simulink model "QuadPIDv2"  (R2024b)
settings: Solver=VariableStepAuto  StartTime=0.0  StopTime=50  RelTol=1e-3
libraries: aerolibutil x9, matrix_library x2, sharedutil x2, sharedtransform x1, simulink_extras x1
settings Model: Creator=Jorge  LastModifiedBy=Jorge

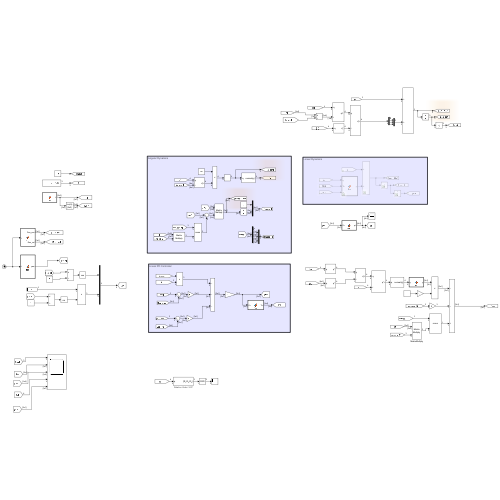
[thumbnail: Simulink's stored preview of the top-level diagram]
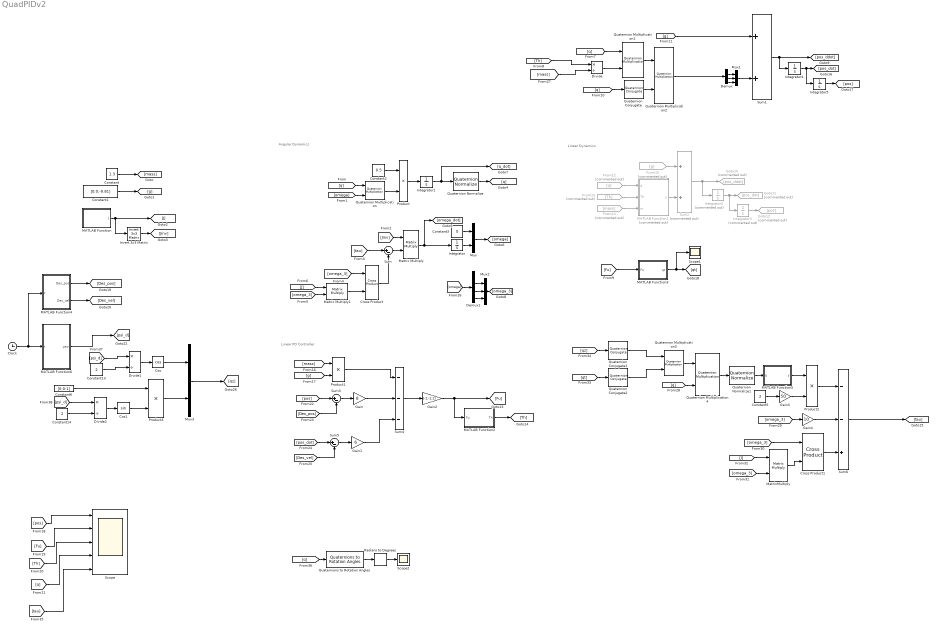
== system QuadPIDv2 ==
  note: Linear PD Controller
  note: Linear Dynamics
  note: Angular Dynamics
  Clock : Clock
  Constant : Constant  Value=1.3
  Constant1 : Constant  Value=[0;0;-9.81]
  Constant13 : Constant  Value=2
  Constant14 : Constant  Value=2
  Constant2 : Constant  Value=0.5
  Constant3 : Constant  Value=0
  Constant5 : Constant  Value=2
  Constant6 : Constant  Value=[0;0;1]
  Cos : Trigonometry  Operator=cos
  Cos1 : Trigonometry
  Cross Product : matrix_library/Cross Product
  Cross Product1 : matrix_library/Cross Product
  Demux : Demux
  Demux1 : Demux
  Divide : Product  Inputs=*/
  Divide1 : Product  Inputs=*/
  Divide2 : Product  Inputs=*/
  From12 : From  Commented=on  GotoTag=q
  From13 : From  Commented=on  GotoTag=Th
  From14 : From  Commented=on  GotoTag=mass
  From15 : From  Commented=on  GotoTag=g
  Gain : Gain  Gain=8
  Gain1 : Gain  Gain=6
  Gain2 : Gain  Gain=[-1;-1;1]
  Gain3 : Gain  Gain=50
  Gain4 : Gain  Gain=10
  Goto10 : Goto  Commented=on  GotoTag=pos_ddot
  Goto11 : Goto  Commented=on  GotoTag=pos_dot
  Goto12 : Goto  Commented=on  GotoTag=pos
  Integrator : Integrator  InitialCondition=[0;0;0]
  Integrator1 : Integrator  InitialCondition=[1;0;0;0]
  Integrator2 : Integrator  Commented=on
  Integrator3 : Integrator  Commented=on
  Integrator4 : Integrator  InitialCondition=[0;0;0]
  Integrator5 : Integrator  InitialCondition=[0;0;0]
  Invert 3x3 Matrix : aerolibutil/Invert  3x3 Matrix
  MATLAB Function : MATLAB Function  TreatAsAtomicUnit=on
  MATLAB Function1 : MATLAB Function  Commented=on  TreatAsAtomicUnit=on
  MATLAB Function2 : MATLAB Function  TreatAsAtomicUnit=on
  MATLAB Function3 : MATLAB Function  TreatAsAtomicUnit=on
  MATLAB Function4 : MATLAB Function  TreatAsAtomicUnit=on
  MATLAB Function5 : MATLAB Function  TreatAsAtomicUnit=on
  MATLAB Function6 : MATLAB Function  TreatAsAtomicUnit=on
  Matrix Multiply : Product  Multiplication=Matrix(*)
  Matrix Multiply1 : Product  Multiplication=Matrix(*)
  MatrixMultiply : Product  Multiplication=Matrix(*)
  Mux : Mux  Inputs=2
  Mux1 : Mux  Inputs=3
  Mux2 : Mux  Inputs=3
  Mux3 : Mux  Inputs=2
  Product{,1..3} (4 alike) : Product
  Quaternion Conjugate : aerolibutil/Quaternion Conjugate
  Quaternion Conjugate1 : aerolibutil/Quaternion Conjugate
  Quaternion Conjugate2 : aerolibutil/Quaternion Conjugate
  Quaternion Multiplication{,1..4} (5 alike) : aerolibutil/Quaternion Multiplication
  Quaternion Normalize : sharedutil/Quaternion Normalize  aMode=aMode
  Quaternion Normalize1 : sharedutil/Quaternion Normalize  aMode=aMode
  Quaternions to Rotation Angles : sharedtransform/Quaternions to Rotation Angles  rotationOrder=XYZ  aMode=aMode
  Radians to Degrees : simulink_extras/Transformations/Radians to Degrees
  Scope : Scope  NumInputPorts=5
  Scope1 : Scope
  Scope2 : Scope
  Sum : Sum  Inputs=|+-
  Sum1 : Sum
  Sum2 : Sum  Commented=on
  Sum3 : Sum  Inputs=|+-
  Sum4 : Sum  Inputs=---
  Sum5 : Sum  Inputs=|+-
  Sum6 : Sum  Inputs=--+
  wires:
  Constant/1 -> [mass]
  Constant1/1 -> [g]
  MATLAB Function/1(J) -> [J], Invert 3x3 Matrix/1
  Invert 3x3 Matrix/1 -> [Jinv]
  Constant2/1 -> Product/1
  [q] -> Quaternion Multiplication/1
  [omega] -> Quaternion Multiplication/2
  Quaternion Multiplication/1 -> Product/2
  Product/1 -> Integrator1/1
  Integrator1/1 -> Quaternion Normalize/1, [q_dot]
  [Jinv] -> Matrix Multiply/1
  Matrix Multiply1/1 -> Cross Product/2
  [omega_3] -> Matrix Multiply1/2
  [J] -> Matrix Multiply1/1
  [omega_3] -> Cross Product/1
  [tau] -> Sum/1
  Cross Product/1 -> Sum/2
  Sum/1 -> Matrix Multiply/2
  Matrix Multiply/1 -> Integrator/1, [omega_dot]
  Constant3/1 -> Mux/1
  Integrator/1 -> Mux/2
  Mux/1 -> [omega]
  Quaternion Normalize/1 -> [q]
  [q] -> Quaternion Multiplication1/1
  [q] -> Quaternion Conjugate/1
  Quaternion Multiplication1/1 -> Quaternion Multiplication2/1
  Quaternion Conjugate/1 -> Quaternion Multiplication2/2
  [g] -> Sum1/1
  From12/1 -> MATLAB Function1/1(q)
  From13/1 -> MATLAB Function1/2(Th)
  From14/1 -> MATLAB Function1/3(m)
  MATLAB Function1/1(y) -> Sum2/2
  Sum2/1 -> Integrator2/1, Goto10/1
  Integrator2/1 -> Integrator3/1, Goto11/1
  Integrator3/1 -> Goto12/1
  From15/1 -> Sum2/1
  [g] -> Product1/2
  Demux/2 -> Mux1/1
  Demux/3 -> Mux1/2
  Demux/4 -> Mux1/3
  Mux1/1 -> Sum1/2
  [pos] -> Scope/1
  [Fu] -> Scope/2
  [Th] -> Scope/3
  [q] -> Scope/4
  Integrator4/1 -> [pos_dot], Integrator5/1
  Integrator5/1 -> [pos]
  Sum4/1 -> Gain2/1
  Product1/1 -> Sum4/1
  MATLAB Function2/1(Th) -> [Th]
  [mass] -> Product1/1
  [Fu] -> MATLAB Function3/1(Fu)
  MATLAB Function3/1(qt) -> Scope1/1, [qt]
  MATLAB Function4/1(Des_pos) -> [Des_pos]
  MATLAB Function4/2(Des_vel) -> [Des_vel]
  [pos] -> Sum3/1
  [Des_pos] -> Sum3/2
  Sum3/1 -> Gain/1
  Gain/1 -> Sum4/2
  Sum5/1 -> Gain1/1
  [pos_dot] -> Sum5/1
  Gain1/1 -> Sum4/3
  [Des_vel] -> Sum5/2
  Gain2/1 -> MATLAB Function2/1(Fu), [Fu]
  [qz] -> Quaternion Conjugate1/1
  [qt] -> Quaternion Conjugate2/1
  Quaternion Multiplication3/1 -> Quaternion Multiplication4/1
  [q] -> Quaternion Multiplication4/2
  Quaternion Multiplication4/1 -> Quaternion Normalize1/1
  Constant5/1 -> Gain3/1
  Gain3/1 -> Product2/2
  MATLAB Function5/1(y) -> Product2/1
  [omega_3] -> Gain4/1
  Product2/1 -> Sum6/1
  Gain4/1 -> Sum6/2
  [omega_3] -> Cross Product1/1
  [J] -> MatrixMultiply/1
  MatrixMultiply/1 -> Cross Product1/2
  [omega_3] -> MatrixMultiply/2
  Cross Product1/1 -> Sum6/3
  Quaternion Conjugate1/1 -> Quaternion Multiplication3/1
  Quaternion Conjugate2/1 -> Quaternion Multiplication3/2
  Mux2/1 -> [omega_3]
  Demux1/3 -> Mux2/2
  Demux1/2 -> Mux2/1
  Demux1/4 -> Mux2/3
  [omega] -> Demux1/1
  Quaternion Normalize1/1 -> MATLAB Function5/1(q)
  Divide/1 -> Quaternion Multiplication1/2
  [Th] -> Divide/1
  [mass] -> Divide/2
  Quaternion Multiplication2/1 -> Demux/1
  Mux3/1 -> [qz]
  Cos/1 -> Mux3/1
  Constant14/1 -> Divide2/2
  Clock/1 -> MATLAB Function4/1(t), MATLAB Function6/1(t)
  [psi_d] -> Divide1/1
  Divide1/1 -> Cos/1
  [psi_d] -> Divide2/1
  Product3/1 -> Mux3/2
  Divide2/1 -> Cos1/1
  Constant13/1 -> Divide1/2
  Cos1/1 -> Product3/2
  Constant6/1 -> Product3/1
  MATLAB Function6/1(yaw) -> [psi_d]
  [tau] -> Scope/5
  [q] -> Quaternions to Rotation Angles/1
  Quaternions to Rotation Angles/1 -> Radians to Degrees/1
  Radians to Degrees/1 -> Scope2/1
  Sum6/1 -> [tau]
  Sum1/1 -> Integrator4/1, [pos_ddot]

== matlab function QuadPIDv2/MATLAB Function ==
  data: J output
function J = fcn()

Jxx = 0.177;
Jyy = 0.177;
Jzz = 0.354; 

J = diag([Jxx,Jyy,Jzz]);

== matlab function QuadPIDv2/MATLAB Function2 ==
  data: Fu input; Th output
function Th = fcn(Fu)

Th = [0 0 0 norm(Fu)];

== matlab function QuadPIDv2/MATLAB Function3 ==
  data: Fu input; qt output
function qt = fcn(Fu)

nz = [0;0;1];

Re = sqrt((1 + dot(Fu/norm(Fu),nz))/2);

vec = cross((Fu/norm(Fu)),nz);

vector = vec/norm(vec);
if norm(vec) ~= 0
    Im = (vec/norm(vec)) * sqrt((1 - dot(Fu/norm(Fu),nz))/2);
else
    Im = [0;0;0] * sqrt((1 - dot(Fu/norm(Fu),nz))/2);
end

qt = [Re;Im];

== matlab function QuadPIDv2/MATLAB Function4 ==
  data: Des_pos output; Des_vel output; t input
function [Des_pos, Des_vel] = fcn(t)

r = 2;
Des_pos = [1;1;1];
%Des_pos = [r*cos(1*t) + r;r*sin(1*t);.1*t];
%Des_pos = [1;r*sin(0.1*t);1];
%Des_pos = [r*cos(t);r*sin(t);1];
Des_vel = [0;0;0];

== matlab function QuadPIDv2/MATLAB Function5 ==
  data: q input; y output
function y = fcn(q)

q = q/norm(q);

q_0 = q(1);
q_1 = q(2);
q_2 = q(3);
q_3 = q(4);

w = norm(q);

v = [q_1 q_2 q_3];
v_norm = norm(v);
angle = acos(q_0/w);

if v_norm == 0
    im = [0 0 0];
else
    im = [0 0 0];
    im = (v/v_norm)* acos(q_0);
end

y = transpose([im]);

== matlab function QuadPIDv2/MATLAB Function6 ==
  data: yaw output; t input
function yaw = fcn(t)

flag = 0;
if flag == 0
    yaw = 1* t;
else
    yaw = -1 * t;
end

if yaw == pi
    flag = 1;
end


%yaw = pi;

== matlab function QuadPIDv2/MATLAB Function1 ==
  data: q input; y output; Th input; m input
function y = fcn(q,Th,m)

q = transpose(q);

q1 = quatmultiply(q,(Th/m));
q2 = quatmultiply(q1,quatconj(q));

y = [q2(2);q2(3);q2(4)];
